simulink model "step4"  (Simulink 7.9)
settings: Solver=ode45  StartTime=0.0  StopTime=10.0  RelTol=1e-3
values from neighbouring files (symbols this model uses):
  A = [0.8 0.3; 0 -0.6]    [setup.m]
  P = dlyap(A',Q)    [setup.m]
  x0 = [1;-0.5]    [setup.m]
libraries: simulink x2
settings Model: Creator=aeagr  LastModifiedBy=aeagr

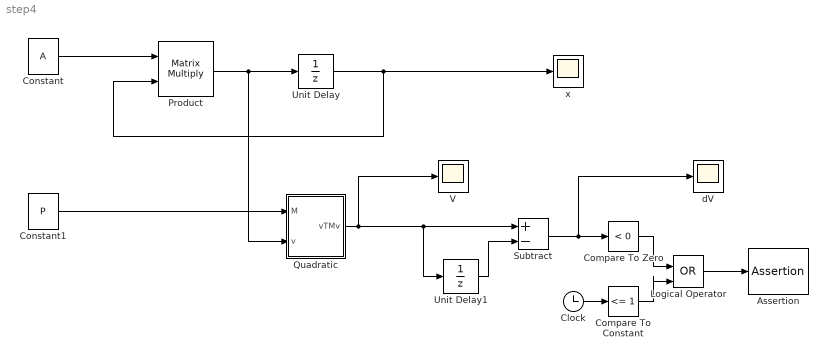
== system step4 ==
  Assertion : Assertion  Enabled=on
  Clock : Clock
  Compare To Constant : simulink/Logic and Bit Operations/Compare To Constant  relop=<=  const=1  OutDataTypeStr=boolean
  Compare To Zero : simulink/Logic and Bit Operations/Compare To Zero  relop=<  OutDataTypeStr=boolean
  Constant : Constant  Value=A
  Constant1 : Constant  Value=P
  Logical Operator : Logic  Operator=OR  IconShape=distinctive  AllPortsSameDT=off  OutDataTypeStr=boolean
  Product : Product  Multiplication=Matrix(*)  RndMeth=Zero
  Quadratic : Subsystem
  Subtract : Sum  Inputs=+-
  Unit Delay : UnitDelay  X0=x0
  Unit Delay1 : UnitDelay
  V : Scope
      settings: SaveName=ScopeData2
  dV : Scope
  x : Scope
  wires:
  Constant/1 -> Product/1
  Product/1 -> Quadratic/2(v), Unit Delay/1
  Unit Delay/1 -> Product/2, x/1
  Constant1/1 -> Quadratic/1(M)
  Quadratic/1(vTMv) -> V/1, Unit Delay1/1, Subtract/1
  Unit Delay1/1 -> Subtract/2
  Subtract/1 -> Compare To Zero/1, dV/1
  Clock/1 -> Compare To Constant/1
  Logical Operator/1 -> Assertion/1
  Compare To Zero/1 -> Logical Operator/1
  Compare To Constant/1 -> Logical Operator/2

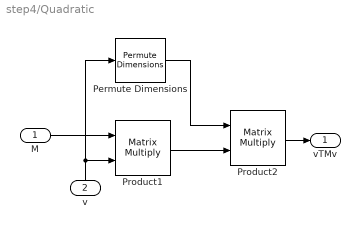
== system step4/Quadratic ==
  M : Inport
  v : Inport  Port=2
  Permute Dimensions : PermuteDimensions
  Product1 : Product  Multiplication=Matrix(*)  RndMeth=Zero
  Product2 : Product  Multiplication=Matrix(*)  RndMeth=Zero
  vTMv : Outport
  wires:
  Product1/1 -> Product2/2
  Permute Dimensions/1 -> Product2/1
  v/1 -> Product1/2, Permute Dimensions/1
  M/1 -> Product1/1
  Product2/1 -> vTMv/1
